simulink model "Project3Week1_notireslip"  (R2024b)
settings: Solver=VariableStepAuto  StartTime=0.0  StopTime=765  RelTol=1e-3
values from neighbouring files (symbols this model uses):
  ad = 2.25    [Project3Week1.m]
  cd = 0.34    [Project3Week1.m]
  ipt = 10    [Project3Week1.m]
  iw = 9    [Project3Week1.m]
  kd = .005    (= 0.005)    [Project3Week1.m]
  ki = .02    (= 0.02)    [Project3Week1.m]
  kp = 0.0075    [Project3Week1.m]
  l_time = l_time(2:end)    [Project3Week1.m]
  l_vel = l_vel(2:end) * 0.44704    [Project3Week1.m]
  rho = 1.293    [Project3Week1.m]
  rw = 0.48/2    (= 0.24)    [Project3Week1.m]
  tau_max = 1600    [Project3Week1.m]
  vm = 1600    [Project3Week1.m]
settings Model: Creator=btagl  LastModifiedBy=btagl

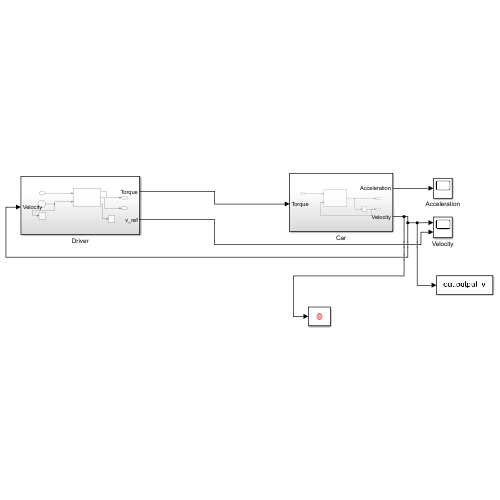
[thumbnail: Simulink's stored preview of the top-level diagram]
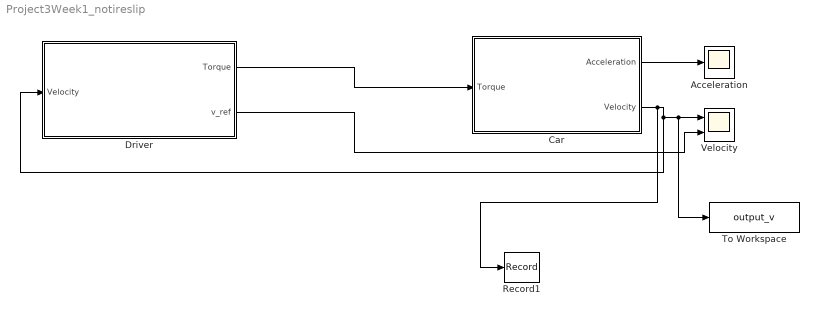
== system Project3Week1_notireslip ==
  Acceleration : Scope
  Car : Subsystem
  Driver : Subsystem
  Record1 : Record  VariableName=actual_v  RecordToWorkspace=on  FileSettingsInternal="{\"entries\":[{\"content\":{\"excelSettings\":{\"content\":{},\"type\":\"Streamout.ExcelSettings\"}},\"type\":\"Streamout.FileSettingStorage\",\"uuid\":\"\"}],\"packageUris\":[\"http:\\/\\/schema.mathworks.com\\/mf0\\/streamout_blocks\\/R2020a\"],\"version\":\"1.0\"}"  SignalsInternal="{\"entries\":[{\"content\":{\"signals\":[{\"content\":{\"blockPath\":[],\"dimensions\":[1],\"domain\":\"\",\"lineColor\":\"#4dbeee\",\"lineWidth\":2,\"plots\":[ 1 ],\"port\":1,\"sid\":[\"\"],\"signalID\":1,\"signalName\":\"Subsystem:2\"},\"type\":\"RecordBlkView.Signal\",\"uuid\":\"\"}]},\"type\":\"RecordBlkView.InputSignals\",\"uuid\":\"\"}],\"packageUris\":[\"http:\\/\\/schema.mathworks.com\\/mf0\\/streamout_blocks\\/R2020a\"],\"version\":\"1.0\"}"  VisualizationBindings="{\"sparklinesplugin\":{\"info\":[{\"bindingParametersList\":[],\"subplotID\":1}]}}"
  To Workspace : ToWorkspace  VariableName=output_v  SampleTime=-1
  Velocity : Scope  NumInputPorts=2
  wires:
  Driver/1(Torque) -> Car/1(Torque)
  Car/2(Velocity) -> Record1/1, To Workspace/1, Velocity/1, Driver/1(Velocity)
  Car/1(Acceleration) -> Acceleration/1
  Driver/2(v_ref) -> Velocity/2

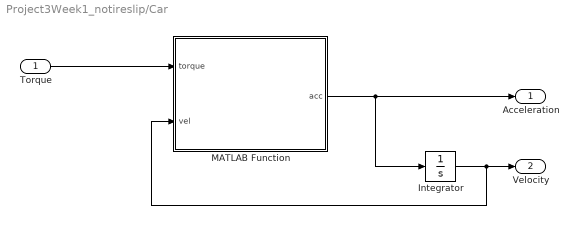
== system Project3Week1_notireslip/Car ==
  Torque : Inport
  Integrator : Integrator
  MATLAB Function : MATLAB Function  TreatAsAtomicUnit=on
  Acceleration : Outport
  Velocity : Outport  Port=2
  wires:
  Torque/1 -> MATLAB Function/1(torque)
  MATLAB Function/1(acc) -> Integrator/1, Acceleration/1
  Integrator/1 -> MATLAB Function/2(vel), Velocity/1

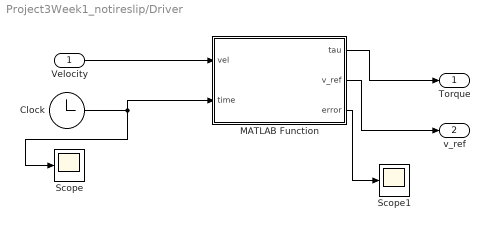
== system Project3Week1_notireslip/Driver ==
  Velocity : Inport
  Clock : Clock
  MATLAB Function : MATLAB Function  TreatAsAtomicUnit=on
  Scope : Scope
  Scope1 : Scope
  Torque : Outport
  v_ref : Outport  Port=2
  wires:
  Velocity/1 -> MATLAB Function/1(vel)
  MATLAB Function/1(tau) -> Torque/1
  Clock/1 -> Scope/1, MATLAB Function/2(time)
  MATLAB Function/2(v_ref) -> v_ref/1
  MATLAB Function/3(error) -> Scope1/1

== matlab function Project3Week1_notireslip/Driver/MATLAB Function ==
  settings: updateMethod=DISCRETE  sampleTime=0.001
  data: vel input; tau output; tau_max parameter; time input; l_time parameter; l_vel parameter; v_ref output; error output; kp parameter; ki parameter; kd parameter
function [tau,v_ref,error]= driver_model(vel, tau_max,time,l_time,l_vel,kp, ki, kd)

    
    % Persistent variables for integral and previous error
    persistent integral_error prev_error;
    if isempty(integral_error)
        integral_error = 0;
        prev_error = 0;
    end
    
    v_ref = interp1(l_time, l_vel, time, 'linear', 'extrap');    % Compute error
    error = v_ref - vel;
    
    % PID Controller
    integral_error = integral_error + error;
    derivative_error = error - prev_error;
    prev_error = error;
    
    alpha_driver = kp * error + ki * integral_error + kd * derivative_error;
    
    % Limit to [-1, 1]
    alpha_driver = max(-1, min(1, alpha_driver));

    % Compute torque
    tau = alpha_driver * tau_max;
end

== matlab function Project3Week1_notireslip/Car/MATLAB Function ==
  data: acc output; torque input; ipt parameter; iw parameter; rw parameter; vm parameter; cd parameter; vel input; ad parameter; rho parameter
function acc = fcn(torque, ipt, iw, rw, vm, cd,vel,ad,rho)

fdrag=0.5*(rho*ad*cd*vel^2);
meq=((ipt+iw)/rw^2)+vm;
fx=(torque/rw)-fdrag;
acc=(fx/meq);
